simulink model "ex7"  (R2020a)
settings: Solver=VariableStepAuto  StartTime=0.0  StopTime=30  RelTol=1e-8
undefined symbols (not defined in the file): A, B, C, D, lambda, x01, x02
settings Model: Creator=Tomo  LastModifiedBy=Tomo

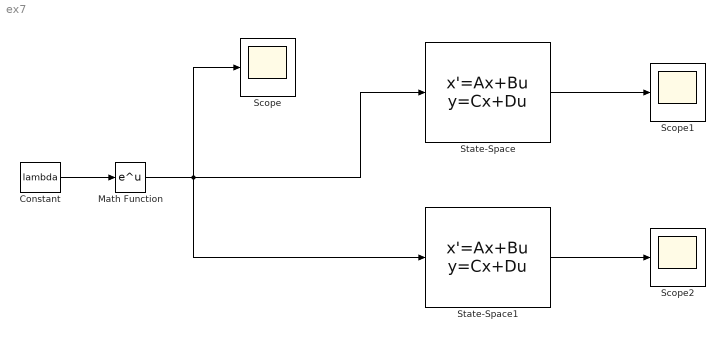
== system ex7 ==
  Constant : Constant  Value=lambda
  Math Function : Math  SaturateOnIntegerOverflow=on
  Scope : Scope
  Scope1 : Scope
  Scope2 : Scope
  State-Space : StateSpace  A=A  B=B  C=C  D=D  InitialCondition=x01
  State-Space1 : StateSpace  A=A  B=B  C=C  D=D  InitialCondition=x02
  wires:
  State-Space/1 -> Scope1/1
  State-Space1/1 -> Scope2/1
  Constant/1 -> Math Function/1
  Math Function/1 -> State-Space1/1, State-Space/1, Scope/1
